simulink model "ButtonLogicTH"  (R2023b)
settings: Solver=VariableStepAuto  StartTime=0.0  StopTime=inf  RelTol=1e-3
settings Model: DataDictionary=ButtonLogicData.sldd  Creator=pkpam  LastModifiedBy=pkpam

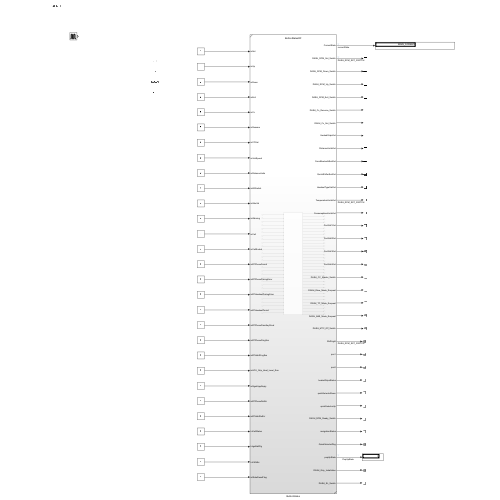
[thumbnail: Simulink's stored preview of the top-level diagram]
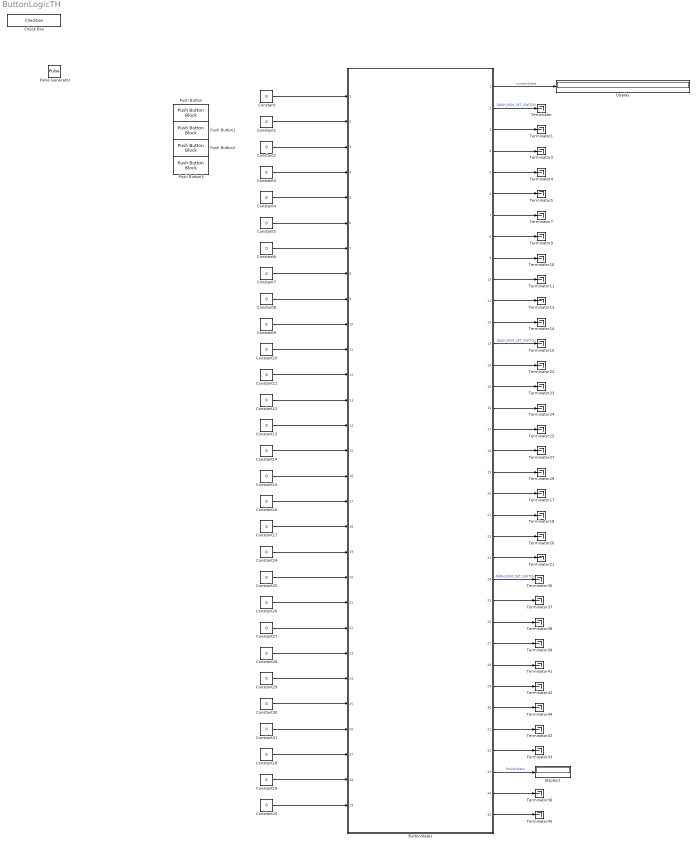
== system ButtonLogicTH ==
  ButtonStates : Subsystem  ReferencedSubsystem=ButtonStatesRF
      settings: PermitHierarchicalResolution=None
  Check Box : Checkbox  LabelPosition=Hide  ShowInitialText=on  Label=ECU_SL_LED
  Constant{,1..20,24..31} (29 alike) : Constant  Value=0  OutDataTypeStr=Inherit: Inherit via back propagation
  Display : Display
  Display1 : Display
  Pulse Generator : DiscretePulseGenerator  PulseType=Time based  Period=10  PulseWidth=5
  Push Button : PushButtonBlock  ButtonText=SET  OffValue=0.000000
  Push Button1 : PushButtonBlock  ButtonText=UP
  Push Button2 : PushButtonBlock  ButtonText=DOWN
  Push Button3 : PushButtonBlock  ButtonText=EXIT
  Terminator{,1,3..5,7,9..11,13..15,17..18,20..25,27,29..30,32..33,36..39,41..42,44..45} (33 alike) : Terminator
  wires:
  Constant/1 -> ButtonStates/1
  ButtonStates/1 -> Display/1  "currentState"
  ButtonStates/2 -> Terminator/1  "DASH_RCM_SET_SWITCH"
  ButtonStates/3 -> Terminator1/1
  ButtonStates/4 -> Terminator3/1
  ButtonStates/7 -> Terminator7/1
  ButtonStates/6 -> Terminator5/1
  ButtonStates/5 -> Terminator4/1
  ButtonStates/10 -> Terminator11/1
  ButtonStates/11 -> Terminator13/1
  ButtonStates/12 -> Terminator14/1
  ButtonStates/9 -> Terminator10/1
  ButtonStates/8 -> Terminator9/1
  ButtonStates/21 -> Terminator18/1
  ButtonStates/20 -> Terminator17/1
  ButtonStates/17 -> Terminator25/1
  ButtonStates/23 -> Terminator21/1
  ButtonStates/16 -> Terminator24/1
  ButtonStates/18 -> Terminator27/1
  ButtonStates/22 -> Terminator20/1
  ButtonStates/13 -> Terminator15/1  "DASH_RCM_SET_SWITCH"
  ButtonStates/14 -> Terminator22/1
  ButtonStates/19 -> Terminator29/1
  ButtonStates/15 -> Terminator23/1
  ButtonStates/32 -> Terminator33/1
  ButtonStates/31 -> Terminator32/1
  ButtonStates/28 -> Terminator41/1
  ButtonStates/34 -> Terminator36/1
  ButtonStates/27 -> Terminator39/1
  ButtonStates/29 -> Terminator42/1
  ButtonStates/33 -> Display1/1  "PopUpState"
  ButtonStates/24 -> Terminator30/1  "DASH_RCM_SET_SWITCH"
  ButtonStates/25 -> Terminator37/1
  ButtonStates/30 -> Terminator44/1
  ButtonStates/26 -> Terminator38/1
  ButtonStates/35 -> Terminator45/1
  Constant1/1 -> ButtonStates/2
  Constant2/1 -> ButtonStates/3
  Constant3/1 -> ButtonStates/4
  Constant4/1 -> ButtonStates/5
  Constant5/1 -> ButtonStates/6
  Constant6/1 -> ButtonStates/7
  Constant7/1 -> ButtonStates/8
  Constant8/1 -> ButtonStates/9
  Constant9/1 -> ButtonStates/10
  Constant10/1 -> ButtonStates/11
  Constant11/1 -> ButtonStates/12
  Constant12/1 -> ButtonStates/13
  Constant13/1 -> ButtonStates/14
  Constant14/1 -> ButtonStates/15
  Constant15/1 -> ButtonStates/16
  Constant16/1 -> ButtonStates/17
  Constant17/1 -> ButtonStates/18
  Constant24/1 -> ButtonStates/19
  Constant25/1 -> ButtonStates/20
  Constant26/1 -> ButtonStates/21
  Constant27/1 -> ButtonStates/22
  Constant28/1 -> ButtonStates/23
  Constant29/1 -> ButtonStates/24
  Constant30/1 -> ButtonStates/25
  Constant31/1 -> ButtonStates/26
  Constant18/1 -> ButtonStates/27
  Constant19/1 -> ButtonStates/28
  Constant20/1 -> ButtonStates/29
